simulink model "HVDCVSCBased"  (R2024b)
settings: Solver=ode45  StartTime=0.0  StopTime=3  FixedStep=Ts_Power  RelTol=1e-3  AbsTol=1e-2
InitFcn:
  | Fnom = 50;        % Hz
  | 
  | Fc = 27*Fnom;   % (Hz)
  | Ts_Power = 1/(Fc*100);
  | Ts_Control = Ts_Power*10;
undefined symbols (not defined in the file or in its folder): D1, Delta, DiscIntNeverNeededParam, magnitude
libraries: spsSecondOrderFilterLib x20, spsSeriesRLCBranchLib x14, spsMeanVariableFrequencyLib x12, spsabctoAlphaBetaZeroLib x8, spsThreePhaseVIMeasurementLib x6, spsAlphaBetaZerotodq0Lib x6, spsCurrentMeasurementLib x4, spsThreePhaseHarmonicFilterLib x4, spsVoltageMeasurementLib x4, spsFirstOrderFilterLib x4, spsGroundLib x3, spsThreePhaseSeriesRLCBranchLib x3
(part 1 of 5)
Description:
  | The 'Model  initialization function' defined in the
  | 
  | Model Properties automatically sets the sample time
  | 
  | Ts to 50e-6 s
settings Model: Creator=The MathWorks, Inc.  LastModifiedBy=prankfarsons
settings SolverCC: AutoScaleAbsTol=off  AlgebraicLoopSolver=TrustRegion
settings DataIOCC: SaveFormat=StructureWithTime  SaveTime=off  ReturnWorkspaceOutputs=off  SignalLoggingName=sigsOut
settings OptimizationCC: BlockReduction=off  BooleanDataType=off  ExpressionDepthLimit=2147483647  InitFltsAndDblsToZero=on  LifeSpan=inf
settings DebuggingCC: SaveWithParameterizedLinksMsg=none  UnderspecifiedInitializationDetection=Classic  MergeDetectMultiDrivingBlocksExec=none  CheckExecutionContextPreStartOutputMsg=on  SignalResolutionControl=TryResolveAllWithWarning  MultiTaskDSMMsg=warning  MultiTaskCondExecSysMsg=none  FcnCallInpInsideContextMsg=warning  StateNameClashWarn=warning  SFUnexpectedBacktrackingDiag=warning  SFNoUnconditionalDefaultTransitionDiag=warning  SFExecutionAtInitializationDiag=none  ArithmeticOperatorsInVariantConditions=warning
settings HardwareCC: ProdBitPerPointer=32  ProdBitPerSizeT=32  ProdBitPerPtrDiffT=32  ProdLargestAtomicFloat=None  ProdIntDivRoundTo=Undefined  ProdEndianess=Unspecified  ProdWordSize=32  ProdHWDeviceType=32-bit Generic  TargetHWDeviceType=32-bit Generic  ProdEqTarget=off
settings ModelReferenceCC: EnableRefExpFcnMdlSchedulingChecks=on  PropagateSignalLabelsOutOfModel=off
settings SFSimCC: SimUseLocalCustomCode=off  CustomCodeUndefinedFunction=UseInterfaceOnly
settings RTWCC: RTWUseLocalCustomCode=off  GPUComputeCapability=3.5  DLArmComputeVersion=19.05
settings CodeAppCC: StateflowObjectComments=on
settings GRTTargetCC: TargetFcnLib=ansi_tfl_tmw.mat  TargetLangStandard=C89/C90 (ANSI)  CombineOutputUpdateFcns=off  GRTInterface=on
settings ConfigComp: CovMetricSettings=dw  CovSaveCumulativeToWorkspaceVar=on  CovSaveSingleToWorkspaceVar=on  CovExternalEMLEnable=off  CovSFcnEnable=off
settings SimscapeCC: SimscapeNormalizeSystem=off

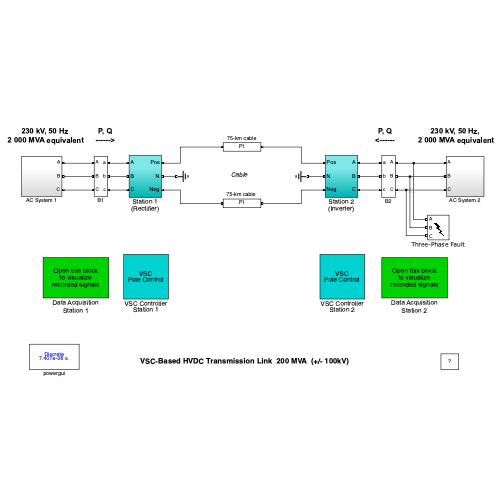
[thumbnail: Simulink's stored preview of the top-level diagram]
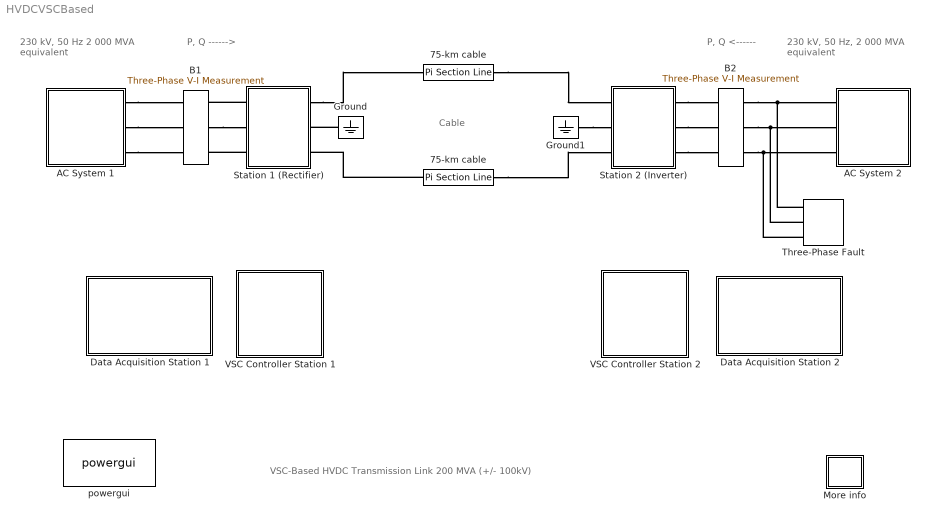
== system HVDCVSCBased ==
  note: VSC-Based HVDC Transmission Link 200 MVA (+/- 100kV)
  note: 230 kV, 50 Hz,
      | 2 000 MVA equivalent
  note: Cable
  note: P, Q
      | ------>
  note: P, Q
      | <------
  note: 230 kV, 50 Hz
      |  2 000 MVA equivalent
  75-km cable : spsPiSectionLineLib/Pi Section Line  LConnTagsString=__new0  RConnTagsString=__new0  Phases=1  PiSections=2  Length=75  Frequency=Fnom  Resistance=1.3900e-002  Inductance=1.5900e-004  Capacitance=2.3100e-007  SpecifyConductance=off  Conductance=0  Measurements=None  Measurements2=None
  "75-km cable " : spsPiSectionLineLib/Pi Section Line  LConnTagsString=__new0  RConnTagsString=__new0  Phases=1  PiSections=2  Length=75  Frequency=Fnom  Resistance=1.3900e-002  Inductance=1.5900e-004  Capacitance=2.3100e-007  SpecifyConductance=off  Conductance=0  Measurements=None  Measurements2=None
  AC System 1 : Subsystem
  AC System 2 : Subsystem
  B1 : spsThreePhaseVIMeasurementLib/Three-Phase V-I Measurement  VoltageMeasurement=phase-to-ground  SetLabelV=on  LabelV=Uabc_B1  Vpu=on  VpuLL=off  CurrentMeasurement=yes  SetLabelI=on  LabelI=Iabc_B1  Ipu=on  Pbase=200e6  Vbase=230e3  OutputType=Magnitude  PhasorSimulation=off  PSBequivalent=0
  B2 : spsThreePhaseVIMeasurementLib/Three-Phase V-I Measurement  VoltageMeasurement=phase-to-ground  SetLabelV=on  LabelV=Uabc_B2  Vpu=on  VpuLL=off  CurrentMeasurement=yes  SetLabelI=on  LabelI=Iabc_B2  Ipu=on  Pbase=200e6  Vbase=230e3  OutputType=Magnitude  PhasorSimulation=off  PSBequivalent=0
  Data Acquisition Station 1 : Subsystem
      mask Display: disp('Open this block\nto visualize\nrecorded signals')
  Data Acquisition Station 2 : Subsystem
      mask Display: disp('Open this block\nto visualize\nrecorded signals')
  Ground : spsGroundLib/Ground  LConnTagsString=a
  Ground1 : spsGroundLib/Ground  LConnTagsString=a
  More info : Subsystem
      settings: OpenFcn="showExample(\"simscapeelectricalsps/HVDCVSCBasedExample\")"
      mask Display: disp('?')
  Station 1 (Rectifier) : Subsystem
  Station 2 (Inverter) : Subsystem
  Three-Phase Fault : spsThreePhaseFaultLib/Three-Phase Fault  InitialStates=0  FaultA=on  FaultB=on  FaultC=on  GroundFault=on  SwitchTimes="( [0   0.12] + 2.1)*100"  External=off  SwitchStatus=NaN  FaultResistance=0.001  GroundResistance=0.001  SnubberResistance=1e6  SnubberCapacitance=inf  Measurements=None
  VSC Controller Station 1 : Subsystem
      mask Display: disp('VSC\nPole Control')
  VSC Controller Station 2 : Subsystem
      mask Display: disp('VSC\nPole Control')
  powergui : spspowerguiLib/powergui  Priority=2  SimulationMode=Discrete  SampleTime=Ts_Power  frequency=60  Iterations=50  frequencyindice=50  Pbase=100e6  ErrMax=1e-4  UnitsV=kV  UnitsW=MW  buscounter=0  FunctionMessages=off  echomessages=off  EnableUseOfTLC=off  CurrentSourceSwitches=off  DisableSnubberDevices=off  DisableRonSwitches=off  DisableVfSwitches=off  DisplayEquations=off  AutomaticDiscreteSolvers=off  SolverType=Tustin/Backward Euler (TBE)  Interpol=off  ExternalGateDelay=off  methode=off  Ts=0  x0status=blocks  SPID=off  SwTol=0  HookPort=off  NonlinearTolerance=1e-4  nMaxIteration=100  ContinueOnMaxIteration=off  RestoreLinks=warning  ResistiveCurrentMeasurement=off  Frange=[0:2:500]  Ylog=off  Xlog=on  ShowGrid=off  save=off  variable=ZData  structure=res_fft  ZoomFFT=on  StartTime=1.5  cycles=2  DisplayStyle=1  fundamental=50  FreqAxis=off  MaxFrequency=3000  frequencyindicesteady=1  RmsSteady=1  display=off
  connections:
  Station 1 (Rectifier)/LConn1 -- B1/RConn1
  B1/RConn2 -- Station 1 (Rectifier)/LConn2
  Station 1 (Rectifier)/LConn3 -- B1/RConn3
  "75-km cable "/LConn1 -- Station 1 (Rectifier)/RConn3
  75-km cable/RConn1 -- Station 2 (Inverter)/RConn1
  "75-km cable "/RConn1 -- Station 2 (Inverter)/RConn3
  B2/LConn1 -- Three-Phase Fault/LConn1 -- AC System 2/RConn1
  Station 2 (Inverter)/LConn1 -- B2/RConn1
  Station 2 (Inverter)/LConn2 -- B2/RConn2
  Station 2 (Inverter)/LConn3 -- B2/RConn3
  B2/LConn2 -- Three-Phase Fault/LConn2 -- AC System 2/RConn2
  B2/LConn3 -- Three-Phase Fault/LConn3 -- AC System 2/RConn3
  Ground/LConn1 -- Station 1 (Rectifier)/RConn2
  Ground1/LConn1 -- Station 2 (Inverter)/RConn2
  AC System 1/RConn1 -- B1/LConn1
  AC System 1/RConn2 -- B1/LConn2
  AC System 1/RConn3 -- B1/LConn3
  Station 1 (Rectifier)/RConn1 -- 75-km cable/LConn1

== system HVDCVSCBased/AC System 1 ==
  note: phi = 80 (deg) at 1st & 3rd harm.
  note: System 1
  3- Phase Parallel RLC : spsThreePhaseParallelRLCBranchLib/Three-Phase Parallel RLC Branch  LConnTagsString=A|B|C  RConnTagsString=A|B|C  BranchType=RL  Resistance=13.79  Inductance=31.02e-3  Capacitance=1.0  Measurements=None
  Ground2 : spsGroundLib/Ground  LConnTagsString=a
  Three-Phase Programmable Voltage Source : spsThreePhaseProgrammableVoltageSourceLib/Three-Phase Programmable Voltage Source  PositiveSequence="[230e3  0  Fnom]"  VariationEntity=Amplitude  VariationType=Step  VariationTypeAlt=Step  VariationStep=-0.1  VariationRate=10  VariationMagnitude=0.3  VariationFrequency=2  VariationTiming="[0  0.14] + 1.5"  VariationPhaseA=off  Amplitudes=[1 0.8 1.2 1.0]  TimeValues=[0 0.1 0.15 0.2]  HarmonicGeneration=off  HarmonicA="[2 0.10  0  2]"  HarmonicB="[2  0  35 2]"  Timing="[1.2  99]"  BusType=swing  Pref=0  Qref=0  Qmin=-inf  Qmax=inf
  Three-Phase Series RLC Branch : spsThreePhaseSeriesRLCBranchLib/Three-Phase Series RLC Branch  LConnTagsString=A|B|C  RConnTagsString=A|B|C  BranchType=L  Resistance=1.0  Inductance=62.23e-3  Capacitance=1.0  Measurements=None
  A : PMIOPort  Side=Right
  B : PMIOPort  Port=2  Side=Right
  C : PMIOPort  Port=3  Side=Right
  connections:
  A/RConn1 -- 3- Phase Parallel RLC/RConn1
  B/RConn1 -- 3- Phase Parallel RLC/RConn2
  C/RConn1 -- 3- Phase Parallel RLC/RConn3
  Three-Phase Series RLC Branch/RConn2 -- 3- Phase Parallel RLC/LConn2
  Three-Phase Series RLC Branch/RConn1 -- 3- Phase Parallel RLC/LConn1
  Three-Phase Programmable Voltage Source/RConn1 -- Three-Phase Series RLC Branch/LConn1
  Three-Phase Programmable Voltage Source/RConn2 -- Three-Phase Series RLC Branch/LConn2
  Three-Phase Programmable Voltage Source/RConn3 -- Three-Phase Series RLC Branch/LConn3
  Ground2/LConn1 -- Three-Phase Programmable Voltage Source/LConn1
  Three-Phase Series RLC Branch/RConn3 -- 3- Phase Parallel RLC/LConn3

== system HVDCVSCBased/AC System 2 ==
  note: phi = 80 (deg) at 1st & 3rd harm.
  note: System 2
  " 60 Hz 500kV1" : spsThreePhaseSourceLib/Three-Phase Source  InternalConnection=Yg  VoltagePhases=off  Voltage=230e3  PhaseAngle=0  Voltage_phases=[25e3 25e3 25e3]/sqrt(3)  PhaseAngles_phases=[0 -120 +120]  Frequency=Fnom  NonIdealSource=on  SpecifyImpedance=off  Resistance=0  Inductance=62.23e-3  ShortCircuitLevel=0  BaseVoltage=0  XRratio=0  BusType=swing  Pref=0  Qref=0  Prefabc=[10e3, 10e3, 10e3]  Qrefabc=[0, 0, 0]  Qmin=-inf  Qmax=inf
  3- Phase Parallel RLC1 : spsThreePhaseParallelRLCBranchLib/Three-Phase Parallel RLC Branch  LConnTagsString=A|B|C  RConnTagsString=A|B|C  BranchType=RL  Resistance=13.79  Inductance=31.02e-3  Capacitance=1.0  Measurements=None
  A : PMIOPort  Side=Right
  B : PMIOPort  Port=2  Side=Right
  C : PMIOPort  Port=3  Side=Right
  connections:
  " 60 Hz 500kV1"/RConn1 -- 3- Phase Parallel RLC1/LConn1
  " 60 Hz 500kV1"/RConn2 -- 3- Phase Parallel RLC1/LConn2
  " 60 Hz 500kV1"/RConn3 -- 3- Phase Parallel RLC1/LConn3
  A/RConn1 -- 3- Phase Parallel RLC1/RConn1
  B/RConn1 -- 3- Phase Parallel RLC1/RConn2
  C/RConn1 -- 3- Phase Parallel RLC1/RConn3

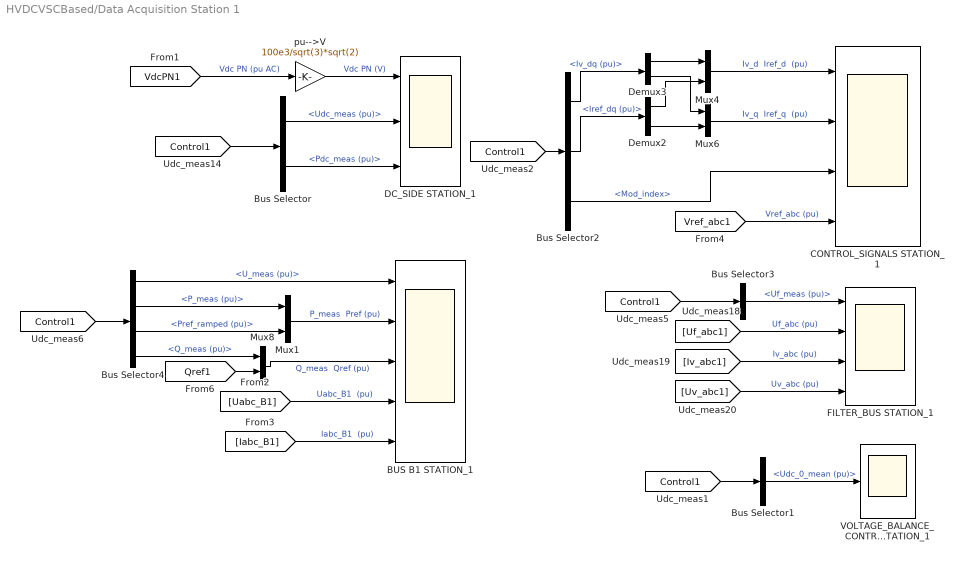
== system HVDCVSCBased/Data Acquisition Station 1 ==
  BUS B1 STATION_1 : Scope  NumInputPorts=5
  Bus Selector : BusSelector  OutputSignals=Udc_meas (pu),Pdc_meas (pu)
  Bus Selector1 : BusSelector  OutputSignals=Udc_0_mean (pu)
  Bus Selector2 : BusSelector  OutputSignals=Iv_dq (pu),Iref_dq (pu),Mod_index
  Bus Selector3 : BusSelector  OutputSignals=Uf_meas (pu)
  Bus Selector4 : BusSelector  OutputSignals=U_meas (pu),P_meas (pu),Pref_ramped (pu),Q_meas (pu)
  "CONTROL_SIGNALS STATION_1 " : Scope  NumInputPorts=4
  DC_SIDE STATION_1 : Scope  NumInputPorts=3
  Demux2 : Demux  Outputs=2
  Demux3 : Demux  Outputs=2
  FILTER_BUS STATION_1 : Scope  NumInputPorts=4
  Mux{1,4,6,8} (4 alike) : Mux  Inputs=2
  VOLTAGE_BALANCE_CONTROL STATION_1 : Scope
  pu-->V : Gain  Gain=100e3/sqrt(3)*sqrt(2)
  wires:
  [VdcPN1] -> pu-->V/1  "Vdc PN (pu AC)"
  Demux3/1 -> Mux4/1
  Demux2/1 -> Mux4/2
  Demux3/2 -> Mux6/1
  Demux2/2 -> Mux6/2
  [Uv_abc1] -> FILTER_BUS STATION_1/4  "Uv_abc (pu)"
  [Iv_abc1] -> FILTER_BUS STATION_1/3  "Iv_abc (pu)"
  [Uf_abc1] -> FILTER_BUS STATION_1/2  "Uf_abc (pu)"
  Bus Selector3/1 -> FILTER_BUS STATION_1/1  "<Uf_meas (pu)>"
  Bus Selector/2 -> DC_SIDE STATION_1/3  "<Pdc_meas (pu)>"
  [Control1] -> Bus Selector/1
  Bus Selector/1 -> DC_SIDE STATION_1/2  "<Udc_meas (pu)>"
  Bus Selector4/1 -> BUS B1 STATION_1/1  "<U_meas (pu)>"
  Bus Selector4/2 -> Mux1/1  "<P_meas (pu)>"
  Bus Selector4/3 -> Mux1/2  "<Pref_ramped (pu)>"
  Bus Selector4/4 -> Mux8/1  "<Q_meas (pu)>"
  [Uabc_B1] -> BUS B1 STATION_1/4  "Uabc_B1  (pu)"
  [Iabc_B1] -> BUS B1 STATION_1/5  "Iabc_B1  (pu)"
  Mux1/1 -> BUS B1 STATION_1/2  "P_meas  Pref (pu)"
  Mux8/1 -> BUS B1 STATION_1/3  "Q_meas  Qref (pu)"
  [Control1] -> Bus Selector2/1
  pu-->V/1 -> DC_SIDE STATION_1/1  "Vdc PN (V)"
  Bus Selector2/1 -> Demux3/1  "<Iv_dq (pu)>"
  Bus Selector2/3 -> "CONTROL_SIGNALS STATION_1 "/3  "<Mod_index>"
  [Control1] -> Bus Selector3/1
  [Control1] -> Bus Selector4/1
  Bus Selector2/2 -> Demux2/1  "<Iref_dq (pu)>"
  [Control1] -> Bus Selector1/1
  Bus Selector1/1 -> VOLTAGE_BALANCE_CONTROL STATION_1/1  "<Udc_0_mean (pu)>"
  Mux4/1 -> "CONTROL_SIGNALS STATION_1 "/1  "Iv_d  Iref_d  (pu)"
  Mux6/1 -> "CONTROL_SIGNALS STATION_1 "/2  "Iv_q  Iref_q  (pu)"
  [Vref_abc1] -> "CONTROL_SIGNALS STATION_1 "/4  "Vref_abc (pu)"
  [Qref1] -> Mux8/2

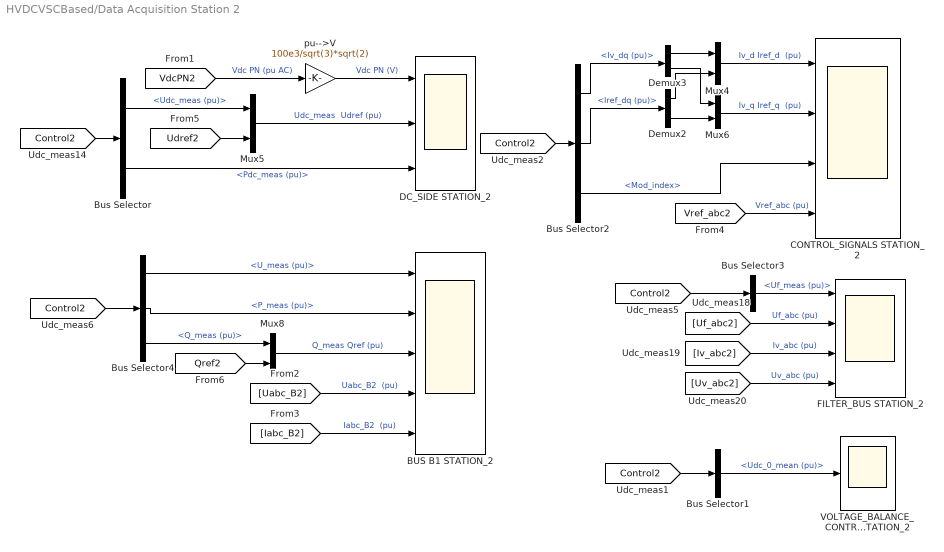
== system HVDCVSCBased/Data Acquisition Station 2 ==
  BUS B1 STATION_2 : Scope  NumInputPorts=5
  Bus Selector : BusSelector  OutputSignals=Udc_meas (pu),Pdc_meas (pu)
  Bus Selector1 : BusSelector  OutputSignals=Udc_0_mean (pu)
  Bus Selector2 : BusSelector  OutputSignals=Iv_dq (pu),Iref_dq (pu),Mod_index
  Bus Selector3 : BusSelector  OutputSignals=Uf_meas (pu)
  Bus Selector4 : BusSelector  OutputSignals=U_meas (pu),P_meas (pu),Q_meas (pu)
  "CONTROL_SIGNALS STATION_2 " : Scope  NumInputPorts=4
  DC_SIDE STATION_2 : Scope  NumInputPorts=3
  Demux2 : Demux  Outputs=2
  Demux3 : Demux  Outputs=2
  FILTER_BUS STATION_2 : Scope  NumInputPorts=4
  Mux{4..6,8} (4 alike) : Mux  Inputs=2
  VOLTAGE_BALANCE_CONTROL STATION_2 : Scope
  pu-->V : Gain  Gain=100e3/sqrt(3)*sqrt(2)
  wires:
  [Qref2] -> Mux8/2
  [Udref2] -> Mux5/2
  [Vref_abc2] -> "CONTROL_SIGNALS STATION_2 "/4  "Vref_abc (pu)"
  Mux6/1 -> "CONTROL_SIGNALS STATION_2 "/2  "Iv_q Iref_q  (pu)"
  Mux4/1 -> "CONTROL_SIGNALS STATION_2 "/1  "Iv_d Iref_d  (pu)"
  Bus Selector1/1 -> VOLTAGE_BALANCE_CONTROL STATION_2/1  "<Udc_0_mean (pu)>"
  [Control2] -> Bus Selector1/1
  Bus Selector2/2 -> Demux2/1  "<Iref_dq (pu)>"
  [Control2] -> Bus Selector4/1
  [Control2] -> Bus Selector3/1
  Bus Selector2/3 -> "CONTROL_SIGNALS STATION_2 "/3  "<Mod_index>"
  Bus Selector2/1 -> Demux3/1  "<Iv_dq (pu)>"
  pu-->V/1 -> DC_SIDE STATION_2/1  "Vdc PN (V)"
  [Control2] -> Bus Selector2/1
  Mux8/1 -> BUS B1 STATION_2/3  "Q_meas Qref (pu)"
  [Iabc_B2] -> BUS B1 STATION_2/5  "Iabc_B2  (pu)"
  [Uabc_B2] -> BUS B1 STATION_2/4  "Uabc_B2  (pu)"
  Bus Selector4/3 -> Mux8/1  "<Q_meas (pu)>"
  Bus Selector4/1 -> BUS B1 STATION_2/1  "<U_meas (pu)>"
  Bus Selector/1 -> Mux5/1  "<Udc_meas (pu)>"
  [Control2] -> Bus Selector/1
  Bus Selector/2 -> DC_SIDE STATION_2/3  "<Pdc_meas (pu)>"
  Bus Selector3/1 -> FILTER_BUS STATION_2/1  "<Uf_meas (pu)>"
  [Uf_abc2] -> FILTER_BUS STATION_2/2  "Uf_abc (pu)"
  [Iv_abc2] -> FILTER_BUS STATION_2/3  "Iv_abc (pu)"
  [Uv_abc2] -> FILTER_BUS STATION_2/4  "Uv_abc (pu)"
  Demux2/2 -> Mux6/2
  Demux3/2 -> Mux6/1
  Demux2/1 -> Mux4/2
  Demux3/1 -> Mux4/1
  [VdcPN2] -> pu-->V/1  "Vdc PN (pu AC)"
  Mux5/1 -> DC_SIDE STATION_2/2  "Udc_meas  Udref (pu)"
  Bus Selector4/2 -> BUS B1 STATION_2/2  "<P_meas (pu)>"

== system HVDCVSCBased/More info ==

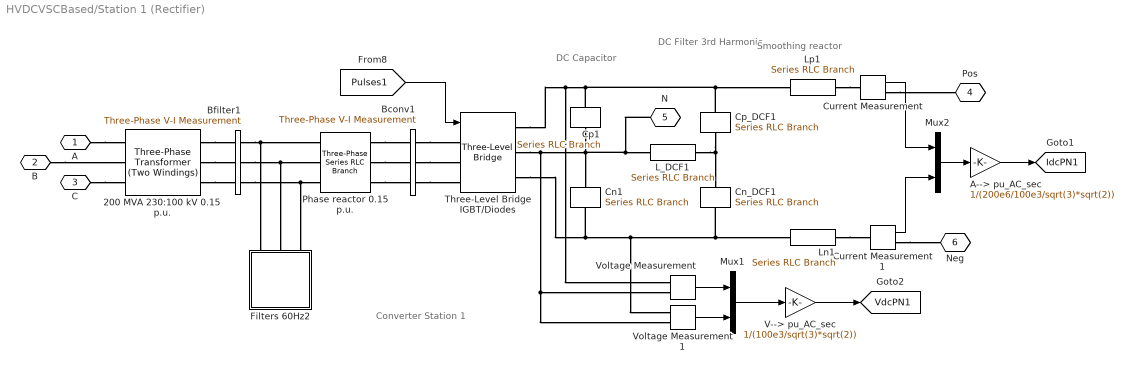
== system HVDCVSCBased/Station 1 (Rectifier) ==
  note: DC Capacitor
  note: Converter Station 1
  note: DC Filter
      | 3rd Harmonic
  note: Smoothing reactor
  200 MVA 230:100 kV 0.15 p.u. : spsThreePhaseTransformerTwoWindingsLib/Three-Phase Transformer (Two Windings)  Winding1Connection=Yg  Winding2Connection=Delta (D1)  CoreType=Three single-phase transformers  SetSaturation=off  Hysteresis=off  DataFile='hysteresis'  SetInitialFlux=off  Measurements=None  UNITS=pu  NominalPower=[200e6 , Fnom]  Winding1="[230e3 * 0.915  0.0025 0.075]"  Winding2="[100e3  0.0025  0.075]"  Rm=500  Lm=500  L0=0.5  Saturation=[ 0,0 ; 0.012,1.25 ; 1.012,1.6 ]  InitialFluxes=[-1.03850588171453 0.527233233676132 0.511272648041703]  BreakLoop=off  DiscreteSolver=Trapezoidal iterative  DataType=off  TransfoNumber=0
  A--> pu_AC_sec : Gain  Gain=1/(200e6/100e3/sqrt(3)*sqrt(2))
  Bconv1 : spsThreePhaseVIMeasurementLib/Three-Phase V-I Measurement  VoltageMeasurement=phase-to-ground  SetLabelV=on  LabelV=Uv_abc1  Vpu=on  VpuLL=off  CurrentMeasurement=yes  SetLabelI=on  LabelI=Iv_abc1  Ipu=on  Pbase=200e6  Vbase=100e3  OutputType=Complex  PhasorSimulation=off  PSBequivalent=0
  Bfilter1 : spsThreePhaseVIMeasurementLib/Three-Phase V-I Measurement  VoltageMeasurement=phase-to-ground  SetLabelV=on  LabelV=Uf_abc1  Vpu=on  VpuLL=off  CurrentMeasurement=no  SetLabelI=off  LabelI=Iabc  Ipu=off  Pbase=100e6  Vbase=100e3  OutputType=Complex  PhasorSimulation=off  PSBequivalent=0
  Cn1 : spsSeriesRLCBranchLib/Series RLC Branch  LConnTagsString=__new0  RConnTagsString=__new0  BranchType=C  Resistance=[]  Inductance=[]  SetiL0=off  InitialCurrent=0  Capacitance=70e-6  Setx0=off  InitialVoltage=0  Measurements=None
  Cn_DCF1 : spsSeriesRLCBranchLib/Series RLC Branch  LConnTagsString=__new0  RConnTagsString=__new0  BranchType=C  Resistance=[]  Inductance=[]  SetiL0=off  InitialCurrent=0  Capacitance=12e-6  Setx0=off  InitialVoltage=0  Measurements=None
  Cp1 : spsSeriesRLCBranchLib/Series RLC Branch  LConnTagsString=__new0  RConnTagsString=__new0  BranchType=C  Resistance=[]  Inductance=[]  SetiL0=off  InitialCurrent=0  Capacitance=70e-6  Setx0=off  InitialVoltage=0  Measurements=None
  Cp_DCF1 : spsSeriesRLCBranchLib/Series RLC Branch  LConnTagsString=__new0  RConnTagsString=__new0  BranchType=C  Resistance=[]  Inductance=[]  SetiL0=off  InitialCurrent=0  Capacitance=12e-6  Setx0=off  InitialVoltage=0  Measurements=None
  Current Measurement : spsCurrentMeasurementLib/Current Measurement  PhasorSimulation=off  OutputType=Complex  PSBequivalent=0
  Current Measurement1 : spsCurrentMeasurementLib/Current Measurement  PhasorSimulation=off  OutputType=Complex  PSBequivalent=0
  Filters 60Hz2 : Subsystem
      mask Display: disp('AC filters\n40 Mvar')
  L_DCF1 : spsSeriesRLCBranchLib/Series RLC Branch  LConnTagsString=__new0  RConnTagsString=__new0  BranchType=RL  Resistance=0.14737  Inductance=46.908e-3  SetiL0=off  InitialCurrent=0  Capacitance=[]  Setx0=off  InitialVoltage=0  Measurements=None
  Ln1 : spsSeriesRLCBranchLib/Series RLC Branch  LConnTagsString=__new0  RConnTagsString=__new0  BranchType=RL  Resistance=0.0251  Inductance=8.0e-3  SetiL0=off  InitialCurrent=0  Capacitance=[]  Setx0=off  InitialVoltage=0  Measurements=Branch current
  Lp1 : spsSeriesRLCBranchLib/Series RLC Branch  LConnTagsString=__new0  RConnTagsString=__new0  BranchType=RL  Resistance=0.0251  Inductance=8.0e-3  SetiL0=off  InitialCurrent=0  Capacitance=[]  Setx0=off  InitialVoltage=0  Measurements=Branch current
  Mux1 : Mux  Inputs=2
  Mux2 : Mux  Inputs=2
  Phase reactor 0.15 p.u. : spsThreePhaseSeriesRLCBranchLib/Three-Phase Series RLC Branch  LConnTagsString=A|B|C  RConnTagsString=A|B|C  BranchType=RL  Resistance=0.0015*(100^2 / 200)  Inductance=0.15* (100^2 / 200) / (2*pi*Fnom)  Capacitance=1.0  Measurements=None
  Three-Level Bridge IGBT/Diodes : spsThreeLevelBridgeLib/Three-Level Bridge  Arms=3  SnubberResistance=5000  SbubberCapacitance=1e-6  Device=IGBT / Diodes  Ron=1e-3  ForwardVoltages="[  0  0  ]"  Measurements=None
  V--> pu_AC_sec : Gain  Gain=1/(100e3/sqrt(3)*sqrt(2))
  Voltage Measurement : spsVoltageMeasurementLib/Voltage Measurement  PhasorSimulation=off  OutputType=Complex  PSBequivalent=0
  Voltage Measurement1 : spsVoltageMeasurementLib/Voltage Measurement  PhasorSimulation=off  OutputType=Complex  PSBequivalent=0
  A : PMIOPort  Side=Left
  B : PMIOPort  Port=2  Side=Left
  C : PMIOPort  Port=3  Side=Left
  Pos : PMIOPort  Tag=PMCPort  Port=4  Side=Right
  N : PMIOPort  Tag=PMCPort  Port=5  Side=Right
  Neg : PMIOPort  Tag=PMCPort  Port=6  Side=Right
  tag scope: IdcPN1=global, VdcPN1=global
  wires:
  [Pulses1] -> Three-Level Bridge IGBT/Diodes/1
  Current Measurement/1 -> Mux2/1
  Current Measurement1/1 -> Mux2/2
  Mux2/1 -> A--> pu_AC_sec/1
  Voltage Measurement/1 -> Mux1/1
  Voltage Measurement1/1 -> Mux1/2
  Mux1/1 -> V--> pu_AC_sec/1
  V--> pu_AC_sec/1 -> [VdcPN1]
  A--> pu_AC_sec/1 -> [IdcPN1]
  connections:
  A/RConn1 -- 200 MVA 230:100 kV 0.15 p.u./LConn1
  B/RConn1 -- 200 MVA 230:100 kV 0.15 p.u./LConn2
  C/RConn1 -- 200 MVA 230:100 kV 0.15 p.u./LConn3
  Phase reactor 0.15 p.u./RConn1 -- Bconv1/LConn1
  Phase reactor 0.15 p.u./RConn2 -- Bconv1/LConn2
  Phase reactor 0.15 p.u./RConn3 -- Bconv1/LConn3
  Bconv1/RConn1 -- Three-Level Bridge IGBT/Diodes/LConn1
  Bconv1/RConn2 -- Three-Level Bridge IGBT/Diodes/LConn2
  Bconv1/RConn3 -- Three-Level Bridge IGBT/Diodes/LConn3
  Cn1/RConn1 -- Three-Level Bridge IGBT/Diodes/RConn3 -- Voltage Measurement1/LConn1 -- Cn_DCF1/RConn1 -- Ln1/LConn1
  Cp_DCF1/LConn1 -- Three-Level Bridge IGBT/Diodes/RConn1 -- Voltage Measurement/LConn1 -- Cp1/LConn1 -- Lp1/LConn1
  Current Measurement/RConn1 -- Pos/RConn1
  Current Measurement1/RConn1 -- Neg/RConn1
  200 MVA 230:100 kV 0.15 p.u./RConn1 -- Bfilter1/LConn1
  200 MVA 230:100 kV 0.15 p.u./RConn2 -- Bfilter1/LConn2
  200 MVA 230:100 kV 0.15 p.u./RConn3 -- Bfilter1/LConn3
  Bfilter1/RConn2 -- Phase reactor 0.15 p.u./LConn2 -- Filters 60Hz2/LConn2
  Bfilter1/RConn3 -- Phase reactor 0.15 p.u./LConn3 -- Filters 60Hz2/LConn3
  Bfilter1/RConn1 -- Phase reactor 0.15 p.u./LConn1 -- Filters 60Hz2/LConn1
  Cp_DCF1/RConn1 -- Cn_DCF1/LConn1 -- L_DCF1/RConn1
  N/RConn1 -- Voltage Measurement/LConn2 -- Voltage Measurement1/LConn2 -- Three-Level Bridge IGBT/Diodes/RConn2 -- Cn1/LConn1 -- Cp1/RConn1 -- L_DCF1/LConn1
  Lp1/RConn1 -- Current Measurement/LConn1
  Ln1/RConn1 -- Current Measurement1/LConn1

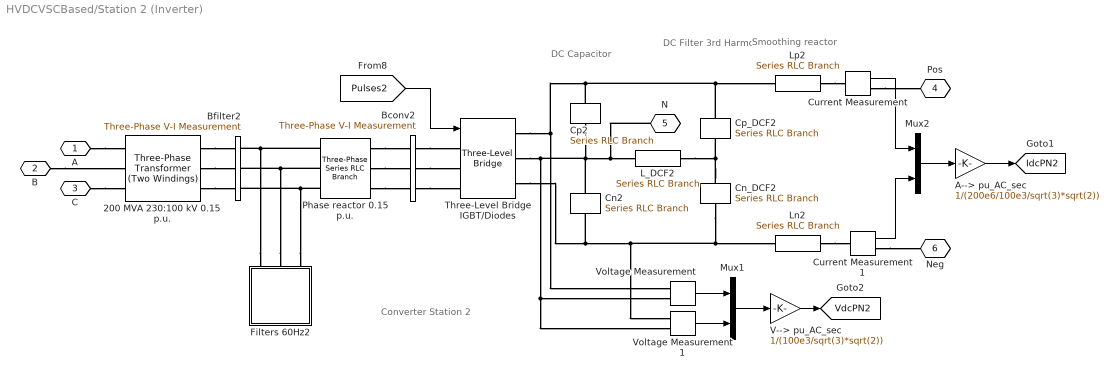
== system HVDCVSCBased/Station 2 (Inverter) ==
  note: Converter Station 2
  note: DC Capacitor
  note: DC Filter
      | 3rd Harmonic
  note: Smoothing reactor
  200 MVA 230:100 kV 0.15 p.u. : spsThreePhaseTransformerTwoWindingsLib/Three-Phase Transformer (Two Windings)  Winding1Connection=Yg  Winding2Connection=Delta (D1)  CoreType=Three single-phase transformers  SetSaturation=off  Hysteresis=off  DataFile='hysteresis'  SetInitialFlux=off  Measurements=None  UNITS=pu  NominalPower=[200e6 , Fnom]  Winding1="[230e3 * 1.015   0.0025  0.075]"  Winding2="[100e3  0.0025  0.075]"  Rm=500  Lm=500  L0=0.5  Saturation=[ 0,0 ; 0.012,1.25 ; 1.012,1.6 ]  InitialFluxes=[-1.00735070526646 0.511416236666093 0.495934468600514]  BreakLoop=off  DiscreteSolver=Trapezoidal iterative  DataType=off  TransfoNumber=0
  A--> pu_AC_sec : Gain  Gain=1/(200e6/100e3/sqrt(3)*sqrt(2))
  Bconv2 : spsThreePhaseVIMeasurementLib/Three-Phase V-I Measurement  VoltageMeasurement=phase-to-ground  SetLabelV=on  LabelV=Uv_abc2  Vpu=on  VpuLL=off  CurrentMeasurement=yes  SetLabelI=on  LabelI=Iv_abc2  Ipu=on  Pbase=200e6  Vbase=100e3  OutputType=Complex  PhasorSimulation=off  PSBequivalent=0
  Bfilter2 : spsThreePhaseVIMeasurementLib/Three-Phase V-I Measurement  VoltageMeasurement=phase-to-ground  SetLabelV=on  LabelV=Uf_abc2  Vpu=on  VpuLL=off  CurrentMeasurement=no  SetLabelI=off  LabelI=Iabc  Ipu=off  Pbase=100e6  Vbase=100e3  OutputType=Complex  PhasorSimulation=off  PSBequivalent=0
  Cn2 : spsSeriesRLCBranchLib/Series RLC Branch  LConnTagsString=__new0  RConnTagsString=__new0  BranchType=C  Resistance=[]  Inductance=[]  SetiL0=off  InitialCurrent=0  Capacitance=70e-6  Setx0=off  InitialVoltage=0  Measurements=None
  Cn_DCF2 : spsSeriesRLCBranchLib/Series RLC Branch  LConnTagsString=__new0  RConnTagsString=__new0  BranchType=C  Resistance=[]  Inductance=[]  SetiL0=off  InitialCurrent=0  Capacitance=12e-6  Setx0=off  InitialVoltage=0  Measurements=None
  Cp2 : spsSeriesRLCBranchLib/Series RLC Branch  LConnTagsString=__new0  RConnTagsString=__new0  BranchType=C  Resistance=[]  Inductance=[]  SetiL0=off  InitialCurrent=0  Capacitance=70e-6  Setx0=off  InitialVoltage=0  Measurements=None
  Cp_DCF2 : spsSeriesRLCBranchLib/Series RLC Branch  LConnTagsString=__new0  RConnTagsString=__new0  BranchType=C  Resistance=[]  Inductance=[]  SetiL0=off  InitialCurrent=0  Capacitance=12e-6  Setx0=off  InitialVoltage=0  Measurements=None
  Current Measurement : spsCurrentMeasurementLib/Current Measurement  PhasorSimulation=off  OutputType=Complex  PSBequivalent=0
  Current Measurement1 : spsCurrentMeasurementLib/Current Measurement  PhasorSimulation=off  OutputType=Complex  PSBequivalent=0
  Filters 60Hz2 : Subsystem
      mask Display: disp('AC filters\n40 Mvar')
  L_DCF2 : spsSeriesRLCBranchLib/Series RLC Branch  LConnTagsString=__new0  RConnTagsString=__new0  BranchType=RL  Resistance=0.14737  Inductance=46.908e-3  SetiL0=off  InitialCurrent=0  Capacitance=[]  Setx0=off  InitialVoltage=0  Measurements=None
  Ln2 : spsSeriesRLCBranchLib/Series RLC Branch  LConnTagsString=__new0  RConnTagsString=__new0  BranchType=RL  Resistance=0.0251  Inductance=8.0e-3  SetiL0=off  InitialCurrent=0  Capacitance=[]  Setx0=off  InitialVoltage=0  Measurements=Branch current
  Lp2 : spsSeriesRLCBranchLib/Series RLC Branch  LConnTagsString=__new0  RConnTagsString=__new0  BranchType=RL  Resistance=0.0251  Inductance=8.0e-3  SetiL0=off  InitialCurrent=0  Capacitance=[]  Setx0=off  InitialVoltage=0  Measurements=Branch current
  Mux1 : Mux  Inputs=2
  Mux2 : Mux  Inputs=2
  Phase reactor 0.15 p.u. : spsThreePhaseSeriesRLCBranchLib/Three-Phase Series RLC Branch  LConnTagsString=A|B|C  RConnTagsString=A|B|C  BranchType=RL  Resistance=(0.15/100)*(100^2 / 200)  Inductance=0.15 * (100^2 / 200) / (2*pi*Fnom)  Capacitance=1.0  Measurements=None
  Three-Level Bridge IGBT/Diodes : spsThreeLevelBridgeLib/Three-Level Bridge  Arms=3  SnubberResistance=5000  SbubberCapacitance=1e-6  Device=IGBT / Diodes  Ron=1e-3  ForwardVoltages="[ 0  0  ]"  Measurements=None
  V--> pu_AC_sec : Gain  Gain=1/(100e3/sqrt(3)*sqrt(2))
  Voltage Measurement : spsVoltageMeasurementLib/Voltage Measurement  PhasorSimulation=off  OutputType=Complex  PSBequivalent=0
  Voltage Measurement1 : spsVoltageMeasurementLib/Voltage Measurement  PhasorSimulation=off  OutputType=Complex  PSBequivalent=0
  A : PMIOPort  Side=Left
  B : PMIOPort  Port=2  Side=Left
  C : PMIOPort  Port=3  Side=Left
  Pos : PMIOPort  Tag=PMCPort  Port=4  Side=Right
  N : PMIOPort  Tag=PMCPort  Port=5  Side=Right
  Neg : PMIOPort  Tag=PMCPort  Port=6  Side=Right
  tag scope: IdcPN2=global, VdcPN2=global
  wires:
  Mux1/1 -> V--> pu_AC_sec/1
  Voltage Measurement1/1 -> Mux1/2
  Voltage Measurement/1 -> Mux1/1
  Mux2/1 -> A--> pu_AC_sec/1
  Current Measurement1/1 -> Mux2/2
  Current Measurement/1 -> Mux2/1
  [Pulses2] -> Three-Level Bridge IGBT/Diodes/1
  A--> pu_AC_sec/1 -> [IdcPN2]
  V--> pu_AC_sec/1 -> [VdcPN2]
  connections:
  Filters 60Hz2/LConn1 -- Bfilter2/RConn1 -- Phase reactor 0.15 p.u./LConn1
  Filters 60Hz2/LConn3 -- Bfilter2/RConn3 -- Phase reactor 0.15 p.u./LConn3
  Filters 60Hz2/LConn2 -- Bfilter2/RConn2 -- Phase reactor 0.15 p.u./LConn2
  200 MVA 230:100 kV 0.15 p.u./RConn3 -- Bfilter2/LConn3
  200 MVA 230:100 kV 0.15 p.u./RConn2 -- Bfilter2/LConn2
  200 MVA 230:100 kV 0.15 p.u./RConn1 -- Bfilter2/LConn1
  Current Measurement1/RConn1 -- Neg/RConn1
  Current Measurement/RConn1 -- Pos/RConn1
  Cp_DCF2/LConn1 -- Three-Level Bridge IGBT/Diodes/RConn1 -- Voltage Measurement/LConn1 -- Cp2/LConn1 -- Lp2/LConn1
  Cn_DCF2/RConn1 -- Voltage Measurement1/LConn1 -- Three-Level Bridge IGBT/Diodes/RConn3 -- Cn2/RConn1 -- Ln2/LConn1
  Cn2/LConn1 -- Voltage Measurement1/LConn2 -- Voltage Measurement/LConn2 -- Three-Level Bridge IGBT/Diodes/RConn2 -- Cp2/RConn1 -- L_DCF2/LConn1 -- N/RConn1
  Bconv2/RConn3 -- Three-Level Bridge IGBT/Diodes/LConn3
  Bconv2/RConn2 -- Three-Level Bridge IGBT/Diodes/LConn2
  Bconv2/RConn1 -- Three-Level Bridge IGBT/Diodes/LConn1
  Phase reactor 0.15 p.u./RConn3 -- Bconv2/LConn3
  Phase reactor 0.15 p.u./RConn2 -- Bconv2/LConn2
  Phase reactor 0.15 p.u./RConn1 -- Bconv2/LConn1
  C/RConn1 -- 200 MVA 230:100 kV 0.15 p.u./LConn3
  B/RConn1 -- 200 MVA 230:100 kV 0.15 p.u./LConn2
  A/RConn1 -- 200 MVA 230:100 kV 0.15 p.u./LConn1
  Cn_DCF2/LConn1 -- Cp_DCF2/RConn1 -- L_DCF2/RConn1
  Lp2/RConn1 -- Current Measurement/LConn1
  Ln2/RConn1 -- Current Measurement1/LConn1

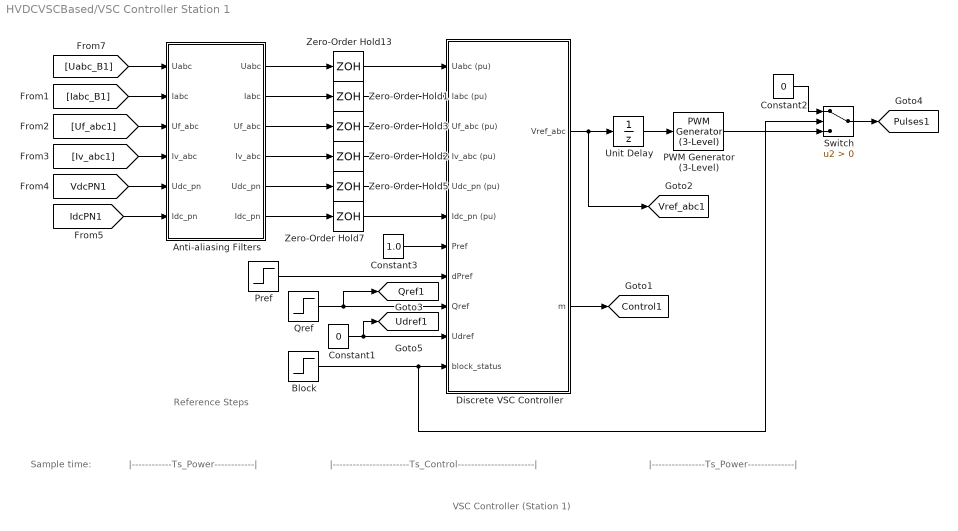
== system HVDCVSCBased/VSC Controller Station 1 ==
  note: |-----------------------Ts_Control-----------------------|
  note: |------------Ts_Power------------|
  note: Sample time:
  note: |----------------Ts_Power--------------|
  note: Reference Steps
  note: VSC Controller
      | (Station 1)
  Anti-aliasing Filters : Subsystem  mask(Anti-aliasing (2nd order lowpass)){f0_aa=2000, Ts=Ts_Power}
      mask prompts: f0_aa "Cut-off frequency (Hz):"; Ts "Sample time:"
      mask init:
      | zeta = 1/sqrt(2);
  Block : Step  Time=0.3  Before=1  After=0  SampleTime=Ts_Control
  Constant1 : Constant  Value=0
  Constant2 : Constant  Value=0
  Constant3 : Constant  Value=1.0
  "Discrete VSC Controller " : Subsystem  mask(Discrete VSC-Based HVDC Controller){Mode=Active & Reactive Power, Xnom=[230e3, 100e3, Fnom, 200e3, 200e6], XP=[20.0, 1.0, -1.0, 1.43], Xdvco=[3.0, 3.0, 1.05, 0.9], XUdc=[2.0, 40.0 ], XQ=[20.0, 0.5, -0.5], Xvco=[3.0, 3.0, 1.05, 0.94], Xcrc=[1.1,  0.8], Xaccc=[0.6, 6.0,  0.3], enable_dcvbc=off, Xdcvbc=[0.2, 0.03], Ts_Control=Ts_Control}
      mask prompts: Mode "Control Mode:"; Xnom "Nominal AC & DC values: [ Vpcc(Vrms L-L) , Vconv (Vrms L-L),  Freq. (Hz), Vdc (V L-L), Pnom (VA) ]"; XP "P Regulator [ Ki (1/s), Pmax (pu), Pmin (pu), Ramp (pu/s)]"; Xdvco "P Control: Udc Override [ Kp, Ki (1/s), Udc_max (pu), Udc_min (pu)]"; XUdc "DC Voltage Regulator [ Kp, Ki (1/s)]"; XQ "Q Regulator [ Ki (1/s), Qmax (pu), Qmin (pu)]"; Xvco "Q Control: Uac Override [ Kp, Ki (1/s), U_max (pu), U_min (pu)]"; Xcrc "Current Reference Limits [ lim_d (pu),  lim_q (pu)]"; Xaccc "Inner Current Regulator [ Kp, Ki (1/s), Kf (pu)]"; enable_dcvbc "DC Voltage Balance"; Xdcvbc "DC Voltage Balance Control} [ Kp, Ki (1/s)]"; Ts_Control "Sample Time (s)"
      mask help:
      | This block implements a controller for a VSC (Voltage-Sourced Converter) HVDC using a three-level or Neutral Point Clamped (NPC) converter bridge.
      | The 'Vref_abc' output contains the three modulating signals used by  the carrier-based  Sinusoidal Pulse Width Modulation (SPWM) pulse generator.
      | The output  'm' is a bus signal . Use the Bus Selector block to extract individual signals.
      |
      | See the "VSC-Based Transmission Link " tutorial for a description of the control system.
      mask init:
      | if (Mode == 1)
      | 	P_control = 1;
      | else
      | 	P_control = 0;
      | end
      | 	
      | % Nominal AC & DC values:
      | VacNom1 = Xnom(1); VacNom2 = Xnom(2); Fnom = Xnom(3);
      | VdcNom = Xnom(4); Pnom = Xnom(5);
      | % Normalisation Calculation
      | Uac_sec_to_pu   = 1/(VacNom2*sqrt(2)/sqrt(3));      % Vrms(L-L) ==> pu Vac
      | k_nom2pu_Vdc = (VdcNom/2) * Uac_sec_to_pu;          % pu Vdc ==> pu Vac    
      | k_pu2nom_Vdc = 1/k_nom2pu_Vdc;                      % pu Vac ==> pu Vdc
      | k_nom2pu_Idc = ((VacNom2)*sqrt(3))/(sqrt(2)*VdcNom);% pu Idc ==> pu Iac
      | k_pu2nom_Idc = 1/k_nom2pu_Idc;                      % pu Iac ==> pu Idc
      | % Transformer connexion:
      | Tr_connection = 1;
      | % P regulator:
      | Ki_apc = XP(1); P_max = XP(2); P_min = XP(3); Ramp_apc = XP(4);
      | max_i_apc = 10; min_i_apc = -max_i_apc; V_level_apc = 0.9;  % (pu)
      | % DC Voltage Control Override:
      | Ki_apc_vco = Xdvco(2); Kp_apc_vco = Xdvco(1);
      | Udc_max = Xdvco(3)*k_nom2pu_Vdc; Udc_min = Xdvco(4)*k_nom2pu_Vdc;
      | max_apc_vco = 1.0; min_apc_vco = -max_apc_vco;
      | % Q regulator:
      | Ki_rpc = XQ(1);Q_max = XQ(2); Q_min = XQ(3);
      | max_i_rpc = 10; min_i_rpc = -max_i_rpc; V_level_rpc = 0.9;  % (pu)
      | % AC Voltage Control Override:
      | Ki_rpc_vco = Xvco(2); Kp_rpc_vco = Xvco(1);
      | U_max = Xvco(3); U_min = Xvco(4);
      | max_rpc_vco = 1.0; min_rpc_vco = -max_rpc_vco;
      | % Current Reference Calculation:
      | lim_d_crc = Xcrc(1); lim_q_crc = Xcrc(2); %(pu)
      | U_level_crc = 0.7; %(pu)
      | f0_crc = 100; % (Hz)
      | % Current Reference Limitation:
      | Iref_max = sqrt(lim_d_crc^2 + lim_q_crc^2);
      | % DC Voltage regulator:
      | Ki_dcvc = XUdc(2); Kp_dcvc = XUdc(1);
      | max_i_dcvc = lim_d_crc; min_i_dcvc = -max_i_dcvc;
      | max_out_dcvc = max_i_dcvc; min_out_dcvc = -max_out_dcvc; % (pu)
      | f0_Udc = 10.0; % (Hz)
      | % Inner Current Loop:
      | Ki_accc = Xaccc(2); Kp_accc = Xaccc(1); Kf_accc = Xaccc(3);
      | max_out_accc = 2.0; min_out_accc = -max_out_accc;
      | %PLL
      | f_min_pll = 0.75*Fnom; % (Hz)
      | Kp_pll = 60.0;
      | Ki_pll = 1400;
      | % Inner Current Loop:
      | K_pwm = 1.0; 
      | % DC Voltage Balance Control:
      | Ki_dcvbc = Xdcvbc(2); Kp_dcvbc = Xdcvbc(1);
      | f0_dcvbc =  1.0;   % (Hz)
      | max_out_dcvbc = 0.2; min_out_dcvbc = -max_out_dcvbc;
      | % Signal Calculations:
      | f0_sc = 17; %(Hz)
      | zeta_sc = 1/sqrt(2);
      mask TypeOptions Mode: Active & Reactive Power | DC Voltage & Reactive  Power
      mask Callback Mode:
      | tempMaskVis=get_param(gcb,'MaskVisibilities');
      | if strcmp(get_param(gcb,'Mode'),'Active & Reactive Power')
      | 	tempMaskVis{2}='on'; tempMaskVis{3}='on'; tempMaskVis{4}='on'; tempMaskVis{5}='on';
      | 	tempMaskVis{6}='on'; tempMaskVis{5}='off'; tempMaskVis{8}='on'; tempMaskVis{9}='on';
      | 	tempMaskVis{10}='on';  tempMaskVis{12}='on';
      | 
      | else
      | 	tempMaskVis{2}='on'; tempMaskVis{3}='off'; tempMaskVis{4}='off'; tempMaskVis{5}='on';
      | 	tempMaskVis{6}='on'; tempMaskVis{7}='on'; tempMaskVis{8}='on'; tempMaskVis{9}='on';
      | 	tempMaskVis{10}='on';  tempMaskVis{12}='on';
      | end
      | if strcmp(get_param(gcb,'enable_dcvbc'),'on')
      | 	tempMaskVis{11}='on';
      | else
      | 	tempMaskVis{11}='off';
      | end
      | set_param(gcb,'MaskVisibilities',tempMaskVis);
      mask Callback enable_dcvbc:
      | tempMaskVis=get_param(gcb,'MaskVisibilities');
      | if strcmp(get_param(gcb,'enable_dcvbc'),'on')
      | 	tempMaskVis{11}='on';
      | else
      | 	tempMaskVis{11}='off';
      | end
      | set_param(gcb,'MaskVisibilities',tempMaskVis);
  PWM Generator (3-Level) : spsPWMGenerator3LevelLib/PWM Generator (3-Level)  ModulatorType=Three-phase bridge (12 pulses)  ModulatorMode=Unsynchronized  nF=27  Fc=27*Fnom  ModulatingSignals=off  m=0.8  Freq=60  Phase=0  Ts=Ts_Power
  Pref : Step  Time=1.5 * 1  After=-0.1  SampleTime=Ts_Control
  Qref : Step  Time=2.0 * 1  After=-0.1  SampleTime=Ts_Control
  Switch : Switch  Criteria=u2 > Threshold  InputSameDT=off
  Unit Delay : UnitDelay  SampleTime=Ts_Control  HasFrameUpgradeWarning=on
  Zero-Order Hold{1..3,5,7,13} (6 alike) : ZeroOrderHold  SampleTime=Ts_Control
  tag scope: Control1=global, Pulses1=global, Qref1=global, Udref1=global, Vref_abc1=global
  wires:
  "Discrete VSC Controller "/1(Vref_abc) -> Unit Delay/1, [Vref_abc1]
  Zero-Order Hold13/1 -> "Discrete VSC Controller "/1(Uabc (pu))
  Zero-Order Hold1/1 -> "Discrete VSC Controller "/2(Iabc (pu))
  Zero-Order Hold3/1 -> "Discrete VSC Controller "/3(Uf_abc (pu))
  Zero-Order Hold2/1 -> "Discrete VSC Controller "/4(Iv_abc (pu))
  Zero-Order Hold5/1 -> "Discrete VSC Controller "/5(Udc_pn (pu))
  Zero-Order Hold7/1 -> "Discrete VSC Controller "/6(Idc_pn (pu))
  [Iabc_B1] -> Anti-aliasing Filters/2("Iabc ")
  [Uf_abc1] -> Anti-aliasing Filters/3("Uf_abc  ")
  [Iv_abc1] -> Anti-aliasing Filters/4("Iv_abc ")
  Anti-aliasing Filters/2(Iabc) -> Zero-Order Hold1/1
  Anti-aliasing Filters/3(Uf_abc) -> Zero-Order Hold3/1
  Anti-aliasing Filters/4(" Iv_abc") -> Zero-Order Hold2/1
  Anti-aliasing Filters/5("Udc_pn ") -> Zero-Order Hold5/1
  Anti-aliasing Filters/6(" Idc_pn") -> Zero-Order Hold7/1
  Unit Delay/1 -> PWM Generator (3-Level)/1
  Switch/1 -> [Pulses1]
  Constant2/1 -> Switch/1
  Constant1/1 -> "Discrete VSC Controller "/10(Udref), [Udref1]
  Qref/1 -> "Discrete VSC Controller "/9(Qref), [Qref1]
  Pref/1 -> "Discrete VSC Controller "/8(dPref)
  Constant3/1 -> "Discrete VSC Controller "/7(Pref)
  Block/1 -> Switch/2, "Discrete VSC Controller "/11(block_status)
  [VdcPN1] -> Anti-aliasing Filters/5("Udc_pn  ")
  [IdcPN1] -> Anti-aliasing Filters/6("Idc_pn ")
  "Discrete VSC Controller "/2(m) -> [Control1]
  [Uabc_B1] -> Anti-aliasing Filters/1("Uabc ")
  Anti-aliasing Filters/1(Uabc) -> Zero-Order Hold13/1
  PWM Generator (3-Level)/1 -> Switch/3

== system HVDCVSCBased/VSC Controller Station 2 ==
  note: VSC Controller
      | (Station 2)
  note: |----------------Ts_Power--------------|
  note: Sample time:
  note: |------------Ts_Power------------|
  note: |---------------------------Ts_Control-------------------------|
  note: Reference Steps
  Anti-aliasing Filters : Subsystem  mask(Anti-aliasing (2nd order lowpass)){f0_aa=2000, Ts=Ts_Power}
      mask prompts: f0_aa "Cut-off frequency (Hz):"; Ts "Sample time:"
      mask init:
      | zeta = 1/sqrt(2);
  Block : Step  Time=0.1  Before=1  After=0  SampleTime=Ts_Control
  Constant1 : Constant  Value=0
  Constant2 : Constant  Value=0
  Constant3 : Constant  Value=0
  Constant4 : Constant  Value=-0.1
  "Discrete VSC Controller " : Subsystem  mask(Discrete VSC-Based HVDC Controller){Mode=DC Voltage & Reactive  Power, Xnom=[230e3, 100e3, Fnom, 200e3, 200e6], XP=[20.0, 1.0, -1.0, 1.43], Xdvco=[3.0, 3.0, 1.05, 0.9], XUdc=[2.0, 40.0 ], XQ=[20.0, 0.5, -0.5], Xvco=[3.0, 3.0, 1.05, 0.94], Xcrc=[1.1,  0.8], Xaccc=[0.6, 6.0,  0.3], enable_dcvbc=on, Xdcvbc=[0.2, 0.03], Ts_Control=Ts_Control}
      mask prompts: Mode "Control Mode:"; Xnom "Nominal AC & DC values: [ Vpcc(Vrms L-L) , Vconv (Vrms L-L),  Freq. (Hz), Vdc (V L-L), Pnom (VA) ]"; XP "P Regulator [ Ki (1/s), Pmax (pu), Pmin (pu), Ramp (pu/s)]"; Xdvco "P Control: Udc Override [ Kp, Ki (1/s), Udc_max (pu), Udc_min (pu)]"; XUdc "DC Voltage Regulator [ Kp, Ki (1/s)]"; XQ "Q Regulator [ Ki (1/s), Qmax (pu), Qmin (pu)]"; Xvco "Q Control: Uac Override [ Kp, Ki (1/s), U_max (pu), U_min (pu)]"; Xcrc "Current Reference Limits [ lim_d (pu),  lim_q (pu)]"; Xaccc "Inner Current Regulator [ Kp, Ki (1/s), Kf (pu)]"; enable_dcvbc "DC Voltage Balance"; Xdcvbc "DC Voltage Balance Control} [ Kp, Ki (1/s)]"; Ts_Control "Sample Time (s)"
      mask help:
      | This block implements a controller for a VSC (Voltage-Sourced Converter) HVDC using a three-level or Neutral Point Clamped (NPC) converter bridge.
      | The 'Vref_abc' output contains the three modulating signals used by  the carrier-based  Sinusoidal Pulse Width Modulation (SPWM) pulse generator.
      | The output  'm' is a bus signal . Use the Bus Selector block to extract individual signals.
      |
      | See the "VSC-Based Transmission Link " tutorial for a description of the control system.
      mask init: same as HVDCVSCBased/VSC Controller Station 1/Discrete VSC Controller 
      mask TypeOptions Mode: Active & Reactive Power | DC Voltage & Reactive  Power
      mask Callback Mode:
      | tempMaskVis=get_param(gcb,'MaskVisibilities');
      | if strcmp(get_param(gcb,'Mode'),'Active & Reactive Power')
      | 	tempMaskVis{2}='on'; tempMaskVis{3}='on'; tempMaskVis{4}='on'; tempMaskVis{5}='on';
      | 	tempMaskVis{6}='on'; tempMaskVis{5}='off'; tempMaskVis{8}='on'; tempMaskVis{9}='on';
      | 	tempMaskVis{10}='on';  tempMaskVis{12}='on';
      | 
      | else
      | 	tempMaskVis{2}='on'; tempMaskVis{3}='off'; tempMaskVis{4}='off'; tempMaskVis{5}='on';
      | 	tempMaskVis{6}='on'; tempMaskVis{7}='on'; tempMaskVis{8}='on'; tempMaskVis{9}='on';
      | 	tempMaskVis{10}='on';  tempMaskVis{12}='on';
      | end
      | if strcmp(get_param(gcb,'enable_dcvbc'),'on')
      | 	tempMaskVis{11}='on';
      | else
      | 	tempMaskVis{11}='off';
      | end
      | set_param(gcb,'MaskVisibilities',tempMaskVis);
      mask Callback enable_dcvbc:
      | tempMaskVis=get_param(gcb,'MaskVisibilities');
      | if strcmp(get_param(gcb,'enable_dcvbc'),'on')
      | 	tempMaskVis{11}='on';
      | else
      | 	tempMaskVis{11}='off';
      | end
      | set_param(gcb,'MaskVisibilities',tempMaskVis);
  PWM Generator (3-Level) : spsPWMGenerator3LevelLib/PWM Generator (3-Level)  ModulatorType=Three-phase bridge (12 pulses)  ModulatorMode=Unsynchronized  nF=27  Fc=27*Fnom  ModulatingSignals=off  m=0.8  Freq=60  Phase=0  Ts=Ts_Power
  Switch : Switch  Criteria=u2 > Threshold  InputSameDT=off
  Udref : Step  Time=2.5 * 1  Before=1.0  After=0.95  SampleTime=Ts_Control
  Unit Delay : UnitDelay  SampleTime=Ts_Control  HasFrameUpgradeWarning=on
  tag scope: Control2=global, Pulses2=global, Qref2=global, Udref2=global, Vref_abc2=global
  wires:
  Block/1 -> Switch/2, "Discrete VSC Controller "/11(block_status)
  Constant2/1 -> Switch/1
  Switch/1 -> [Pulses2]
  Unit Delay/1 -> PWM Generator (3-Level)/1
  [Iv_abc2] -> Anti-aliasing Filters/4("Iv_abc ")
  [Uf_abc2] -> Anti-aliasing Filters/3("Uf_abc  ")
  [Iabc_B2] -> Anti-aliasing Filters/2("Iabc ")
  [Uabc_B2] -> Anti-aliasing Filters/1("Uabc ")
  [VdcPN2] -> Anti-aliasing Filters/5("Udc_pn  ")
  [IdcPN2] -> Anti-aliasing Filters/6("Idc_pn ")
  Anti-aliasing Filters/1(Uabc) -> "Discrete VSC Controller "/1(Uabc (pu))
  Anti-aliasing Filters/2(Iabc) -> "Discrete VSC Controller "/2(Iabc (pu))
  Anti-aliasing Filters/3(Uf_abc) -> "Discrete VSC Controller "/3(Uf_abc (pu))
  Anti-aliasing Filters/4(" Iv_abc") -> "Discrete VSC Controller "/4(Iv_abc (pu))
  Anti-aliasing Filters/5("Udc_pn ") -> "Discrete VSC Controller "/5(Udc_pn (pu))
  Anti-aliasing Filters/6(" Idc_pn") -> "Discrete VSC Controller "/6(Idc_pn (pu))
  Constant3/1 -> "Discrete VSC Controller "/7(Pref)
  Constant4/1 -> "Discrete VSC Controller "/9(Qref), [Qref2]
  Udref/1 -> "Discrete VSC Controller "/10(Udref), [Udref2]
  Constant1/1 -> "Discrete VSC Controller "/8(dPref)
  "Discrete VSC Controller "/2(m) -> [Control2]
  "Discrete VSC Controller "/1(Vref_abc) -> Unit Delay/1, [Vref_abc2]
  PWM Generator (3-Level)/1 -> Switch/3

== system HVDCVSCBased/Station 1 (Rectifier)/Filters 60Hz2 ==
  note: High-pass
      | damped filters
  note: AC Filters, 40 Mvar @ 100 kV
  "27th 18 Mvar Q = 15 " : spsThreePhaseHarmonicFilterLib/Three-Phase Harmonic Filter  LConnTagsString=A|B|C  FilterType=High-pass  FilterConnection=Y (grounded)  ParNom="[100e3  Fnom]"  Qc=40e6 * 0.45  Fr=27*Fnom  Frd=[11*60 13*60]  Q=15  Measurements=None
      settings: AttributesFormatString=\n
  "54th 22 Mvar Q = 15 " : spsThreePhaseHarmonicFilterLib/Three-Phase Harmonic Filter  LConnTagsString=A|B|C  FilterType=High-pass  FilterConnection=Y (grounded)  ParNom="[100e3  Fnom]"  Qc=40e6 * 0.55  Fr=(2*27)*Fnom  Frd=[11*60 13*60]  Q=15  Measurements=None
      settings: AttributesFormatString=\n
  A : PMIOPort  Side=Left
  B : PMIOPort  Port=2  Side=Left
  C : PMIOPort  Port=3  Side=Left
  connections:
  "54th 22 Mvar Q = 15 "/LConn3 -- C/RConn1 -- "27th 18 Mvar Q = 15 "/LConn3
  "54th 22 Mvar Q = 15 "/LConn2 -- B/RConn1 -- "27th 18 Mvar Q = 15 "/LConn2
  "54th 22 Mvar Q = 15 "/LConn1 -- A/RConn1 -- "27th 18 Mvar Q = 15 "/LConn1

== system HVDCVSCBased/Station 2 (Inverter)/Filters 60Hz2 ==
  note: High-pass
      | damped filters
  note: AC Filters, 40 Mvar @ 100 kV
  "27th 18 Mvar Q = 15 " : spsThreePhaseHarmonicFilterLib/Three-Phase Harmonic Filter  LConnTagsString=A|B|C  FilterType=High-pass  FilterConnection=Y (grounded)  ParNom="[100e3  Fnom]"  Qc=40e6 * 0.45  Fr=27*Fnom  Frd=[11*60 13*60]  Q=15  Measurements=None
      settings: AttributesFormatString=\n
  "54th 22 Mvar Q = 15 " : spsThreePhaseHarmonicFilterLib/Three-Phase Harmonic Filter  LConnTagsString=A|B|C  FilterType=High-pass  FilterConnection=Y (grounded)  ParNom=[100e3, Fnom]  Qc=40e6 * 0.55  Fr=(2*27)*Fnom  Frd=[11*60 13*60]  Q=15  Measurements=None
      settings: AttributesFormatString=\n
  A : PMIOPort  Side=Left
  B : PMIOPort  Port=2  Side=Left
  C : PMIOPort  Port=3  Side=Left
  connections:
  "27th 18 Mvar Q = 15 "/LConn3 -- "54th 22 Mvar Q = 15 "/LConn3 -- C/RConn1
  "27th 18 Mvar Q = 15 "/LConn2 -- "54th 22 Mvar Q = 15 "/LConn2 -- B/RConn1
  "27th 18 Mvar Q = 15 "/LConn1 -- "54th 22 Mvar Q = 15 "/LConn1 -- A/RConn1

== system HVDCVSCBased/VSC Controller Station 1/Anti-aliasing Filters ==
  note: Filtering
  note: Low-pass filter
  "Uabc " : Inport  PortDimensions=3
  "Iabc " : Inport  Port=2  PortDimensions=3
  "Uf_abc  " : Inport  Port=3  PortDimensions=3
  "Iv_abc " : Inport  Port=4  PortDimensions=3
  "Udc_pn  " : Inport  Port=5
  "Idc_pn " : Inport  Port=6
  Second-Order Filter{,1..5} (6 alike) : spsSecondOrderFilterLib/Second-Order Filter  FilterType=Lowpass  Fo=f0_aa  Zeta=zeta  Ts=Ts_Control  Initialize=off  Vac_Init="[0,  0,  60]"  Vdc_Init=0  PlotResponse=off  FreqRange=[0, 500, 1]
      settings: AttributesFormatString=f0=%<Fo>
  Uabc : Outport  VectorParamsAs1DForOutWhenUnconnected=off
  Iabc : Outport  Port=2  VectorParamsAs1DForOutWhenUnconnected=off
  Uf_abc : Outport  Port=3  VectorParamsAs1DForOutWhenUnconnected=off
  " Iv_abc" : Outport  Port=4  VectorParamsAs1DForOutWhenUnconnected=off
  "Udc_pn " : Outport  Port=5  VectorParamsAs1DForOutWhenUnconnected=off
  " Idc_pn" : Outport  Port=6  VectorParamsAs1DForOutWhenUnconnected=off
  wires:
  "Iv_abc "/1 -> Second-Order Filter/1
  Second-Order Filter/1 -> " Iv_abc"/1
  "Uf_abc  "/1 -> Second-Order Filter1/1
  Second-Order Filter1/1 -> Uf_abc/1
  "Uabc "/1 -> Second-Order Filter2/1
  Second-Order Filter2/1 -> Uabc/1
  "Udc_pn  "/1 -> Second-Order Filter3/1
  Second-Order Filter3/1 -> "Udc_pn "/1
  "Idc_pn "/1 -> Second-Order Filter4/1
  Second-Order Filter4/1 -> " Idc_pn"/1
  "Iabc "/1 -> Second-Order Filter5/1
  Second-Order Filter5/1 -> Iabc/1
